simulink model "HW1_Moore"  (R2017a)
settings: Solver=FixedStepDiscrete  StartTime=0.0  StopTime=inf  FixedStep=0.0001  RelTol=1e-3  EnableMultiTasking=on
settings Model: Creator=avise  LastModifiedBy=nauga
settings SolverCC: AutoInsertRateTranBlk=on
settings DataIOCC: LimitDataPoints=on
settings OptimizationCC: LifeSpan=inf
settings DebuggingCC: AllowSymbolicDim=off  SFUnexpectedBacktrackingDiag=warning  SFNoUnconditionalDefaultTransitionDiag=warning  SFExecutionAtInitializationDiag=none
settings GRTTargetCC: TargetLangStandard=C89/C90 (ANSI)  GeneratePreprocessorConditionals=Disable all
settings ConfigComp: CovMetricSettings=dw  CovHtmlReporting=on  CovSaveCumulativeToWorkspaceVar=on  CovSaveSingleToWorkspaceVar=on  CovShowResultsExplorer=off  CovExternalEMLEnable=off  CovSFcnEnable=off

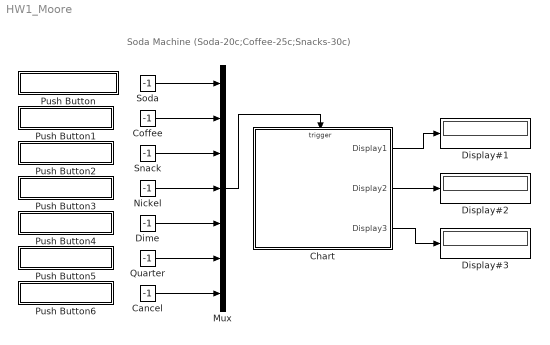
== system HW1_Moore ==
  note: Soda Machine
      | (Soda-20c;Coffee-25c;Snacks-30c)
  Cancel : Constant  Value=-1
  Chart : Stateflow chart  TreatAsAtomicUnit=on
  Coffee : Constant  Value=-1
  Dime : Constant  Value=-1
  Display#1 : Display
  Display#2 : Display
  Display#3 : Display
  Mux : Mux  Inputs=7
  Nickel : Constant  Value=-1
  Push Button : Subsystem  DialogController=hmiCreateDDGDialog  IsWebBlock=on  mask(MWDashboardBlock){webBlockId=664f21db-061d-45c4-a5ed-301e6e3db717, webBlockType=pushbutton, ShowInLibBrwoser=on, ShowInitialText=on, HMISrcModelName=HW1_Moore}
      mask prompts: webBlockId "WebBlock Id"; webBlockType "WebBlock Type"; HMISrcModelName "Source Model"
      mask help: SimulinkHMI:dialogs:PushButtonDialogDesc
      mask Help: helpview([docroot '/mapfiles/simulink.map'], 'hmi_push_button')
      mask Display:
      | model = bdroot(gcb);
      | if strcmp(get_param(model,'BlockDiagramType'), 'library')
      |     image([(matlabroot) '/toolbox/simulink/hmi/icons/PushButton.png']);
      | end
  Push Button1 : Subsystem  DialogController=hmiCreateDDGDialog  IsWebBlock=on  mask(MWDashboardBlock){webBlockId=369ec6e0-de46-472e-8dd1-8918505b40b8, webBlockType=pushbutton, ShowInLibBrwoser=on, ShowInitialText=on, HMISrcModelName=HW1_Moore}
      mask prompts: webBlockId "WebBlock Id"; webBlockType "WebBlock Type"; HMISrcModelName "Source Model"
      mask help: SimulinkHMI:dialogs:PushButtonDialogDesc
      mask Help: helpview([docroot '/mapfiles/simulink.map'], 'hmi_push_button')
      mask Display:
      | model = bdroot(gcb);
      | if strcmp(get_param(model,'BlockDiagramType'), 'library')
      |     image([(matlabroot) '/toolbox/simulink/hmi/icons/PushButton.png']);
      | end
  Push Button2 : Subsystem  DialogController=hmiCreateDDGDialog  IsWebBlock=on  mask(MWDashboardBlock){webBlockId=437ecff1-f85d-43e6-a183-e5cb8b815949, webBlockType=pushbutton, ShowInLibBrwoser=on, ShowInitialText=on, HMISrcModelName=HW1_Moore}
      mask prompts: webBlockId "WebBlock Id"; webBlockType "WebBlock Type"; HMISrcModelName "Source Model"
      mask help: SimulinkHMI:dialogs:PushButtonDialogDesc
      mask Help: helpview([docroot '/mapfiles/simulink.map'], 'hmi_push_button')
      mask Display:
      | model = bdroot(gcb);
      | if strcmp(get_param(model,'BlockDiagramType'), 'library')
      |     image([(matlabroot) '/toolbox/simulink/hmi/icons/PushButton.png']);
      | end
  Push Button3 : Subsystem  DialogController=hmiCreateDDGDialog  IsWebBlock=on  mask(MWDashboardBlock){webBlockId=f2e822cd-a8a7-4ab8-9e8e-7b39c5c413d8, webBlockType=pushbutton, ShowInLibBrwoser=on, ShowInitialText=on, HMISrcModelName=HW1_Moore}
      mask prompts: webBlockId "WebBlock Id"; webBlockType "WebBlock Type"; HMISrcModelName "Source Model"
      mask help: SimulinkHMI:dialogs:PushButtonDialogDesc
      mask Help: helpview([docroot '/mapfiles/simulink.map'], 'hmi_push_button')
      mask Display:
      | model = bdroot(gcb);
      | if strcmp(get_param(model,'BlockDiagramType'), 'library')
      |     image([(matlabroot) '/toolbox/simulink/hmi/icons/PushButton.png']);
      | end
  Push Button4 : Subsystem  DialogController=hmiCreateDDGDialog  IsWebBlock=on  mask(MWDashboardBlock){webBlockId=f0c8a644-454f-4bf4-a778-a88d9125c533, webBlockType=pushbutton, ShowInLibBrwoser=on, ShowInitialText=on, HMISrcModelName=HW1_Moore}
      mask prompts: webBlockId "WebBlock Id"; webBlockType "WebBlock Type"; HMISrcModelName "Source Model"
      mask help: SimulinkHMI:dialogs:PushButtonDialogDesc
      mask Help: helpview([docroot '/mapfiles/simulink.map'], 'hmi_push_button')
      mask Display:
      | model = bdroot(gcb);
      | if strcmp(get_param(model,'BlockDiagramType'), 'library')
      |     image([(matlabroot) '/toolbox/simulink/hmi/icons/PushButton.png']);
      | end
  Push Button5 : Subsystem  DialogController=hmiCreateDDGDialog  IsWebBlock=on  mask(MWDashboardBlock){webBlockId=21d649ba-39b7-4048-9903-c8ade3fb44d4, webBlockType=pushbutton, ShowInLibBrwoser=on, ShowInitialText=on, HMISrcModelName=HW1_Moore}
      mask prompts: webBlockId "WebBlock Id"; webBlockType "WebBlock Type"; HMISrcModelName "Source Model"
      mask help: SimulinkHMI:dialogs:PushButtonDialogDesc
      mask Help: helpview([docroot '/mapfiles/simulink.map'], 'hmi_push_button')
      mask Display:
      | model = bdroot(gcb);
      | if strcmp(get_param(model,'BlockDiagramType'), 'library')
      |     image([(matlabroot) '/toolbox/simulink/hmi/icons/PushButton.png']);
      | end
  Push Button6 : Subsystem  DialogController=hmiCreateDDGDialog  IsWebBlock=on  mask(MWDashboardBlock){webBlockId=33373d40-ddda-4141-b1fc-f71dcaba8225, webBlockType=pushbutton, ShowInLibBrwoser=on, ShowInitialText=on, HMISrcModelName=HW1_Moore}
      mask prompts: webBlockId "WebBlock Id"; webBlockType "WebBlock Type"; HMISrcModelName "Source Model"
      mask help: SimulinkHMI:dialogs:PushButtonDialogDesc
      mask Help: helpview([docroot '/mapfiles/simulink.map'], 'hmi_push_button')
      mask Display:
      | model = bdroot(gcb);
      | if strcmp(get_param(model,'BlockDiagramType'), 'library')
      |     image([(matlabroot) '/toolbox/simulink/hmi/icons/PushButton.png']);
      | end
  Quarter : Constant  Value=-1
  Snack : Constant  Value=-1
  Soda : Constant  Value=-1
  wires:
  Chart/1(Display1) -> Display#1/1
  Chart/2(Display2) -> Display#2/1
  Chart/3(Display3) -> Display#3/1
  Cancel/1 -> Mux/7
  Quarter/1 -> Mux/6
  Dime/1 -> Mux/5
  Nickel/1 -> Mux/4
  Snack/1 -> Mux/3
  Coffee/1 -> Mux/2
  Soda/1 -> Mux/1
  Mux/1 -> Chart/Trigger

== system HW1_Moore/Push Button ==

== system HW1_Moore/Push Button1 ==

== system HW1_Moore/Push Button2 ==

== system HW1_Moore/Push Button3 ==

== system HW1_Moore/Push Button4 ==

== system HW1_Moore/Push Button5 ==

== system HW1_Moore/Push Button6 ==

== stateflow chart HW1_Moore/Chart ==
  state Soda_release
    state Soda_Release1
      en:
      Display2=Display2+5;
      Display3=Display2-20;
      Reset
    state Soda_Release2
      en:
      Display2=Display2+10;
      Display3=Display2-20;
      Reset
    state Soda_Release3
      en:
      Display2=Display2+25;
      Display3=Display2-20;
      Reset
    state Soda_Cancel
      en:
      Display3=Display2;
      Reset
  state Soda
    %20c
    state Soda_Nickel1
      en:
      Display2=Display2+5;
      Display1=1;
    state Soda_Dime
      en:
      Display2=Display2+10;
      Display1=1;
    state Default
    (default) -> Soda.Default
  state Error
    en:
    Display1=9;
  state Wait
    en:
    Display1=0;
    Display2=0;
  state Coffee
    %25c
    state Coffee_Nickel
      en:
      Display2=Display2+5;
      Display1=2;
    state Coffee_Dime
      en:
      Display2=Display2+10;
      Display1=2;
    state Default
    (default) -> Coffee.Default
  state Coffee_release
    state Coffee_Release1
      en:
      Display2=Display2+5;
      Display3=Display2-25;
      Reset
    state Coffee_Release2
      en:
      Display2=Display2+10;
      Display3=Display2-25;
      Reset
    state Coffee_Release3
      en:
      Display2=Display2+25;
      Display3=Display2-25;
      Reset
    state Coffee_Cancel
      en:
      Display3=Display2;
      Reset
  state Error1
    en:
    Display1=9;
  state Snacks_release
    state Snacks_Release1
      en:
      Display2=Display2+5;
      Display3=Display2-30;
      Reset
    state Snacks_Release2
      en:
      Display2=Display2+10;
      Display3=Display2-30;
      Reset
    state Snacks_Release3
      en:
      Display2=Display2+25;
      Display3=Display2-30;
      Reset
    state Snacks_Cancel
      en:
      Display3=Display2;
      Reset
  state Snack
    %30c
    state Snack_Nickel
      en:
      Display2=Display2+5;
      Display1=3;
    state Sonack_Dime
      en:
      Display2=Display2+10;
      Display1=3;
    state Snack_Quarter
      en:
      Display2=Display2+25;
      Display1=3;
    state Default
    (default) -> Snack.Default
  state Error2
    en:
    Display1=9;
  (junction 34) -> Soda_Release1 [order 1] : [Display2+5>=20]
  (junction 45) -> Soda_Release2 [order 2] : [Display2+10>=20]
  Error -> (junction 34) [order 1] : Nickel
  Soda -> (junction 34) [order 1] : Nickel
  (junction 34) -> Soda_Nickel1 [order 2] : [Display2+5<20]
  Error -> (junction 45) [order 2] : Dime
  Soda -> (junction 45) [order 2] : Dime
  (junction 45) -> Soda_Dime [order 1] : [Display2+10<20]
  Wait -> Soda [order 5] : Soda{Display1=1;
      | Display3=-1;}
  Soda -> Error [order 3] : Coffee|Snack
  Error -> Soda_Release3 [order 3] : Quarter
  Soda_release -> (junction 138) : Reset
  Soda -> Soda_Release3 [order 5] : Quarter
  (default) -> Wait
  Soda -> Soda_Cancel [order 4] : Cancel
  (junction 138) -> Wait
  Wait -> Coffee [order 6] : Coffee{Display1=2;
      | Display3=-1;}
  Wait -> Snack [order 7] : Snack{Display1=3;
      | Display3=-1;}
  Coffee -> (junction 78) [order 2] : Nickel
  (junction 78) -> Coffee_Release1 [order 1] : [Display2+5>=25]
  (junction 78) -> Coffee_Nickel [order 2] : [Display2+5<25]
  Error1 -> (junction 78) [order 2] : Nickel
  Coffee_release -> (junction 138) : Reset
  Wait -> Wait [order 1] : Nickel{Display3=5;}
  Wait -> Wait [order 2] : Dime{Display3=10;}
  Wait -> Wait [order 3] : Quarter{Display3=25;}
  Wait -> Wait [order 4] : Cancel
  Snacks_release -> (junction 138) : Reset
  Error1 -> (junction 79) [order 1] : Dime
  Coffee -> (junction 79) [order 1] : Dime
  (junction 79) -> Coffee_Release2 [order 1] : [Display2+10>=25]
  (junction 79) -> Coffee_Dime [order 2] : [Display2+10<25]
  Coffee -> Coffee_Release3 [order 3] : Quarter
  Error1 -> Coffee_Release3 [order 3] : Quarter
  Coffee -> Error1 [order 4] : Soda|Snack
  Coffee -> Coffee_Cancel [order 5] : Cancel
  Error2 -> (junction 93) [order 2] : Nickel
  Snack -> (junction 93) [order 3] : Nickel
  (junction 93) -> Snacks_Release1 [order 1] : [Display2+5>=30]
  (junction 93) -> Snack_Nickel [order 2] : [Display2+5<30]
  Error2 -> (junction 95) [order 1] : Dime
  Snack -> (junction 95) [order 1] : Dime
  (junction 95) -> Snacks_Release2 [order 1] : [Display2+10>=30]
  (junction 95) -> Sonack_Dime [order 2] : [Display2+10<30]
  Snack -> (junction 94) [order 5] : Quarter
  Error2 -> (junction 94) [order 3] : Quarter
  (junction 94) -> Snacks_Release3 [order 1] : [Display2+25>=30]
  (junction 94) -> Snack_Quarter [order 2] : [Display2+25<30]
  Snack -> Error2 [order 4] : Soda|Coffee
  Snack -> Snacks_Cancel [order 2] : Cancel
  data: Display1 output =0; Display2 output =0; Display3 output =-1
  events: Soda input EITHER_EDGE_EVENT; Coffee input EITHER_EDGE_EVENT; Snack input EITHER_EDGE_EVENT; Nickel input RISING_EDGE_EVENT; Dime input RISING_EDGE_EVENT; Quarter input RISING_EDGE_EVENT; Cancel input EITHER_EDGE_EVENT; Reset local FUNCTION_CALL_EVENT
